simulink library "MixerLib"  (R2022b)
settings: Solver=VariableStepAuto  StartTime=0.0  StopTime=10.0  RelTol=1e-3
undefined symbols (not defined in the file or in its folder): maxGain
settings Model: Creator=ak1044356  LastModifiedBy=sa1045272
settings SolverCC: AlgebraicLoopSolver=TrustRegion
settings DebuggingCC: UnconnectedInputMsg=warning  UnconnectedOutputMsg=warning  UnconnectedLineMsg=warning  SFMachineParentedDataDiag=warning  ArithmeticOperatorsInVariantConditions=warning
settings ModelReferenceCC: EnableRefExpFcnMdlSchedulingChecks=on
settings SFSimCC: CustomCodeUndefinedFunction=UseInterfaceOnly

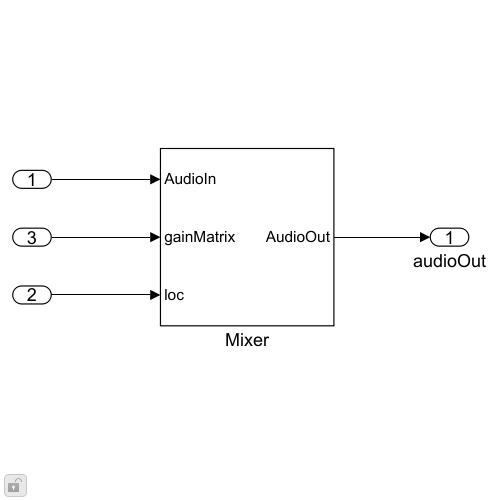
[thumbnail: Simulink's stored preview of the top-level diagram]
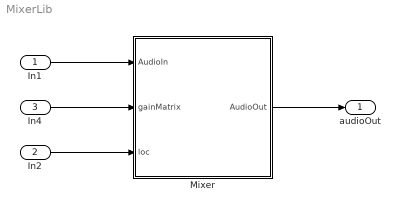
== system MixerLib ==
  In1 : Inport
  In2 : Inport  Port=2
  In4 : Inport  Port=3
  Mixer : Subsystem
  audioOut : Outport  VectorParamsAs1DForOutWhenUnconnected=off
  wires:
  Mixer/1(AudioOut) -> audioOut/1
  In1/1 -> Mixer/1(AudioIn)
  In2/1 -> Mixer/3(loc)
  In4/1 -> Mixer/2(gainMatrix)

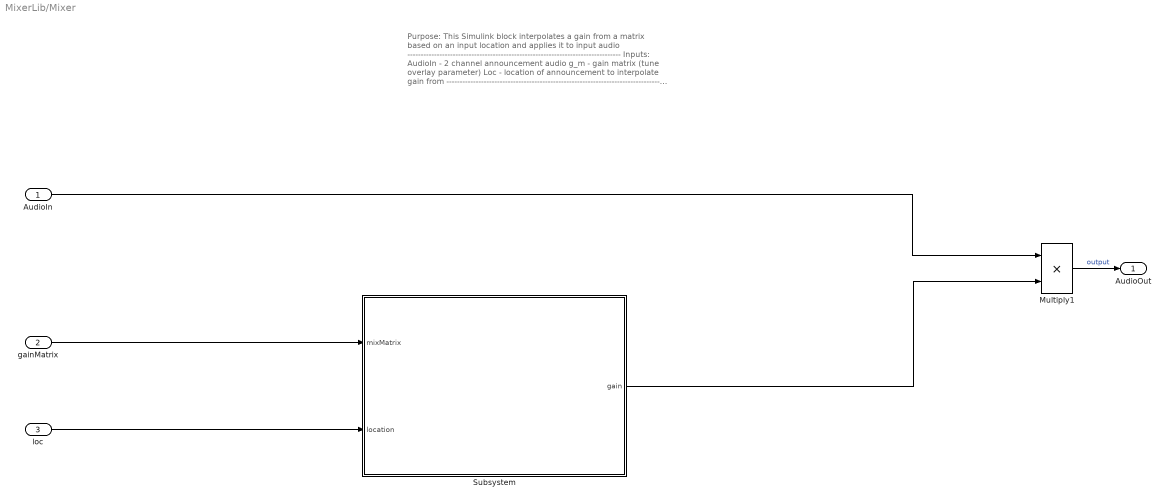
== system MixerLib/Mixer ==
  note: Purpose:
      | This Simulink block interpolates a gain from a matrix
      | based on an input location and applies it to input audio
      | --------------------------------------------------------------------------------
      | Inputs:
      | AudioIn - 2 channel announcement audio
      | g_m - gain matrix (tune overlay parameter)
      | Loc - location of announcement to interpolate gain from
      | --------------------------------------------------------------------------------
      | Outputs:
      | AudioOut - 2 channel announcement audio with applied gain
      | gain [temporary] - gain applied to audio, for debugging
  AudioIn : Inport  OutDataTypeStr=single
  gainMatrix : Inport  Port=2
  loc : Inport  Port=3
  Multiply1 : Product  OutDataTypeStr=single
  Subsystem : Subsystem
  AudioOut : Outport  VectorParamsAs1DForOutWhenUnconnected=off
  wires:
  AudioIn/1 -> Multiply1/1
  Multiply1/1 -> AudioOut/1  "output"
  gainMatrix/1 -> Subsystem/1(mixMatrix)
  Subsystem/1(gain) -> Multiply1/2
  loc/1 -> Subsystem/2(location)

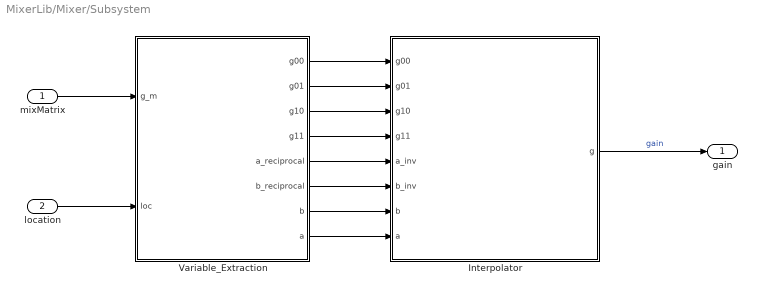
== system MixerLib/Mixer/Subsystem ==
  mixMatrix : Inport
  location : Inport  Port=2
  Interpolator : Subsystem
  Variable_Extraction : Subsystem
  gain : Outport  VectorParamsAs1DForOutWhenUnconnected=off
  wires:
  Interpolator/1(g) -> gain/1  "gain"
  mixMatrix/1 -> Variable_Extraction/1(g_m)
  Variable_Extraction/8(a) -> Interpolator/8(a)
  Variable_Extraction/4(g11) -> Interpolator/4(g11)
  Variable_Extraction/3(g10) -> Interpolator/3(g10)
  Variable_Extraction/2(g01) -> Interpolator/2(g01)
  location/1 -> Variable_Extraction/2(loc)
  Variable_Extraction/5(a_reciprocal) -> Interpolator/5(a_inv)
  Variable_Extraction/1(g00) -> Interpolator/1(g00)
  Variable_Extraction/6(b_reciprocal) -> Interpolator/6(b_inv)
  Variable_Extraction/7(b) -> Interpolator/7(b)

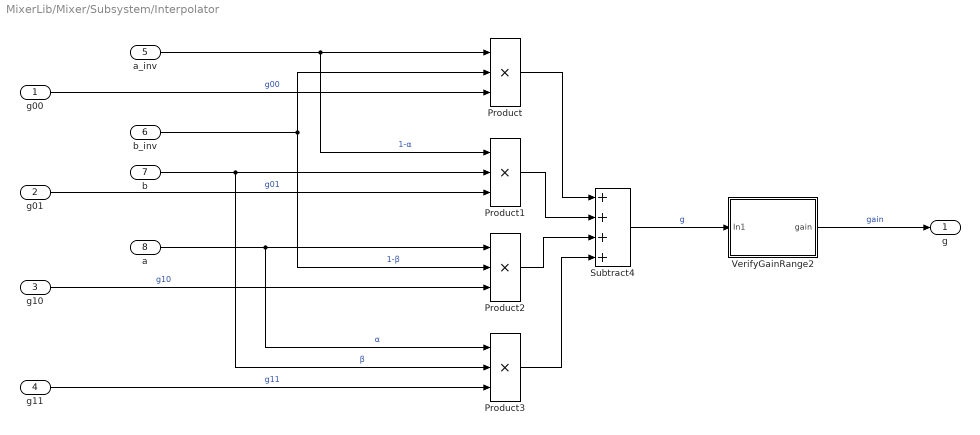
== system MixerLib/Mixer/Subsystem/Interpolator ==
  g00 : Inport
  g01 : Inport  Port=2
  g10 : Inport  Port=3
  g11 : Inport  Port=4
  a_inv : Inport  Port=5
  b_inv : Inport  Port=6
  b : Inport  Port=7
  a : Inport  Port=8
  Product{,1..3} (4 alike) : Product  Inputs=3  OutDataTypeStr=single
  Subtract4 : Sum  Inputs=++++  OutDataTypeStr=single
  VerifyGainRange2 : Subsystem
  g : Outport  VectorParamsAs1DForOutWhenUnconnected=off
  wires:
  g00/1 -> Product/3  "g00"
  Product1/1 -> Subtract4/2
  Product2/1 -> Subtract4/3
  Product3/1 -> Subtract4/4
  a/1 -> Product3/1, Product2/1  "α"
  a_inv/1 -> Product1/1, Product/1  "1-α"
  g10/1 -> Product2/3  "g10"
  b_inv/1 -> Product/2, Product2/2  "1-β"
  Subtract4/1 -> VerifyGainRange2/1(In1)  "g"
  b/1 -> Product1/2, Product3/2  "β"
  Product/1 -> Subtract4/1
  g11/1 -> Product3/3  "g11"
  g01/1 -> Product1/3  "g01"
  VerifyGainRange2/1(gain) -> g/1  "gain"

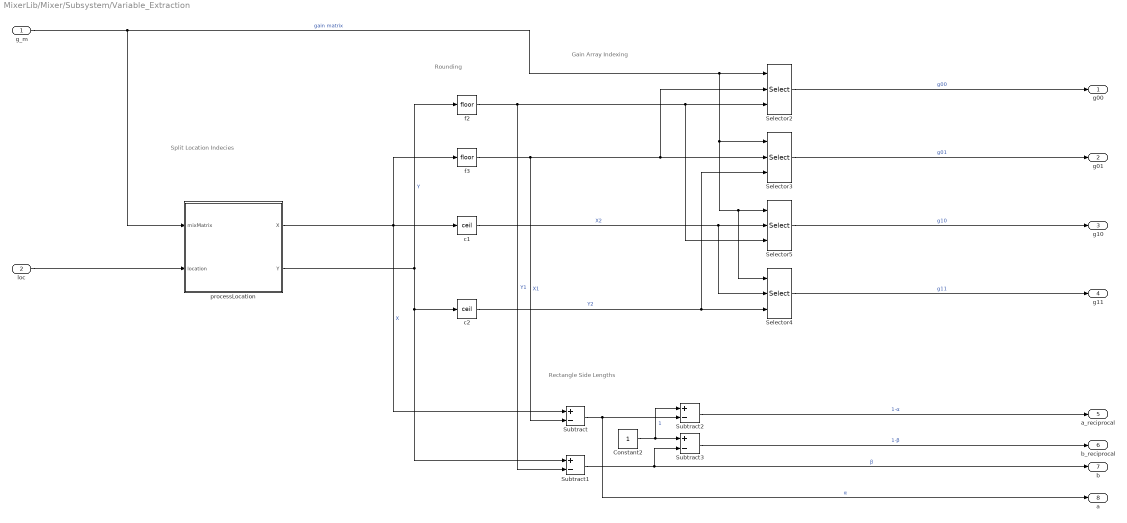
== system MixerLib/Mixer/Subsystem/Variable_Extraction ==
  note: Split Location Indecies
  note: Rectangle Side Lengths
  note: Rounding
  note: Gain Array Indexing
  g_m : Inport  OutDataTypeStr=single
  loc : Inport  Port=2
  Constant2 : Constant  OutDataTypeStr=single
  Selector{2..5} (4 alike) : Selector  NumberOfDimensions=2  InputPortWidth=2  IndexOptions=Index vector (port),Index vector (port)  Indices=[1 3],1  OutputSizes=1,1
  Subtract{,1..3} (4 alike) : Sum  Inputs=+-  OutDataTypeStr=single
  c1 : Rounding  Operator=ceil
  "c2 " : Rounding  Operator=ceil
  f2 : Rounding
  f3 : Rounding
  processLocation : Subsystem
  g00 : Outport  VectorParamsAs1DForOutWhenUnconnected=off
  g01 : Outport  Port=2  VectorParamsAs1DForOutWhenUnconnected=off
  g10 : Outport  Port=3  VectorParamsAs1DForOutWhenUnconnected=off
  g11 : Outport  Port=4  VectorParamsAs1DForOutWhenUnconnected=off
  a_reciprocal : Outport  Port=5  VectorParamsAs1DForOutWhenUnconnected=off
  b_reciprocal : Outport  Port=6  VectorParamsAs1DForOutWhenUnconnected=off
  b : Outport  Port=7  VectorParamsAs1DForOutWhenUnconnected=off
  a : Outport  Port=8  VectorParamsAs1DForOutWhenUnconnected=off
  wires:
  Subtract3/1 -> b_reciprocal/1  "1-β"
  Subtract2/1 -> a_reciprocal/1  "1-α"
  processLocation/2(Y) -> f2/1, Subtract1/1, "c2 "/1  "Y"
  Selector2/1 -> g00/1  "g00"
  Selector3/1 -> g01/1  "g01"
  Selector4/1 -> g11/1  "g11"
  Selector5/1 -> g10/1  "g10"
  Subtract/1 -> a/1, Subtract2/2  "α"
  g_m/1 -> processLocation/1(mixMatrix), Selector4/1, Selector5/1, Selector3/1, Selector2/1  "gain matrix"
  "c2 "/1 -> Selector3/3, Selector4/3  "Y2"
  f2/1 -> Subtract1/2, Selector5/3, Selector2/3  "Y1"
  Constant2/1 -> Subtract2/1, Subtract3/1  "1"
  f3/1 -> Selector3/2, Selector2/2, Subtract/2  "X1"
  c1/1 -> Selector4/2, Selector5/2  "X2"
  Subtract1/1 -> b/1, Subtract3/2  "β"
  processLocation/1(X) -> Subtract/1, f3/1, c1/1  "X"
  loc/1 -> processLocation/2(location)

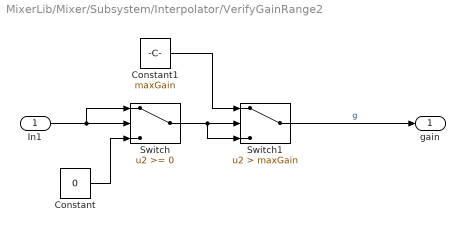
== system MixerLib/Mixer/Subsystem/Interpolator/VerifyGainRange2 ==
  In1 : Inport
  Constant : Constant  Value=0
  Constant1 : Constant  Value=maxGain
  Switch : Switch  SaturateOnIntegerOverflow=off  InputSameDT=off
  Switch1 : Switch  Criteria=u2 > Threshold  Threshold=maxGain  SaturateOnIntegerOverflow=off  InputSameDT=off
  gain : Outport  VectorParamsAs1DForOutWhenUnconnected=off
  wires:
  Switch/1 -> Switch1/3, Switch1/2
  Constant1/1 -> Switch1/1
  In1/1 -> Switch/1, Switch/2
  Switch1/1 -> gain/1  "g"
  Constant/1 -> Switch/3

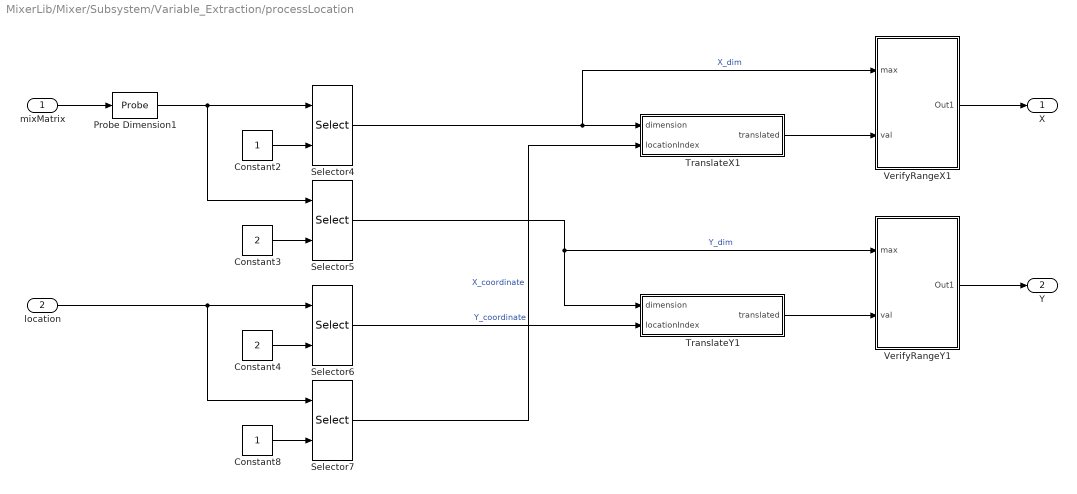
== system MixerLib/Mixer/Subsystem/Variable_Extraction/processLocation ==
  mixMatrix : Inport
  location : Inport  Port=2
  Constant2 : Constant  OutDataTypeStr=single
  Constant3 : Constant  Value=2  OutDataTypeStr=single
  Constant4 : Constant  Value=2  OutDataTypeStr=single
  Constant8 : Constant  OutDataTypeStr=single
  Probe Dimension1 : Probe  ProbeWidth=off  ProbeSampleTime=off  ProbeComplexSignal=off  ProbeSignalDimensions=on
  Selector{4..7} (4 alike) : Selector  InputPortWidth=2  IndexOptions=Index vector (port)  Indices=[1 3]  OutputSizes=1
  TranslateX1 : Subsystem
  TranslateY1 : Subsystem
  VerifyRangeX1 : Subsystem
  VerifyRangeY1 : Subsystem
  X : Outport  VectorParamsAs1DForOutWhenUnconnected=off
  Y : Outport  Port=2  VectorParamsAs1DForOutWhenUnconnected=off
  wires:
  Selector5/1 -> TranslateY1/1(dimension), VerifyRangeY1/1(max)  "Y_dim"
  Selector6/1 -> TranslateY1/2(locationIndex)  "Y_coordinate"
  Selector4/1 -> VerifyRangeX1/1(max), TranslateX1/1(dimension)  "X_dim"
  mixMatrix/1 -> Probe Dimension1/1
  Probe Dimension1/1 -> Selector5/1, Selector4/1
  Selector7/1 -> TranslateX1/2(locationIndex)  "X_coordinate"
  Constant3/1 -> Selector5/2
  location/1 -> Selector7/1, Selector6/1
  Constant4/1 -> Selector6/2
  Constant2/1 -> Selector4/2
  Constant8/1 -> Selector7/2
  TranslateY1/1(translated) -> VerifyRangeY1/2(val)
  TranslateX1/1(translated) -> VerifyRangeX1/2(val)
  VerifyRangeX1/1(Out1) -> X/1
  VerifyRangeY1/1(Out1) -> Y/1

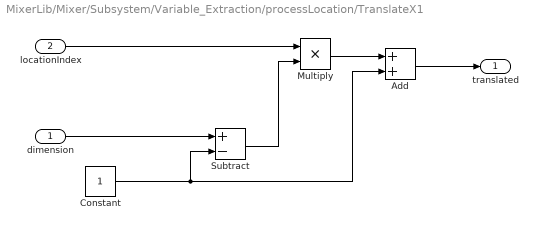
== system MixerLib/Mixer/Subsystem/Variable_Extraction/processLocation/TranslateX1 ==
  dimension : Inport
  locationIndex : Inport  Port=2
  Add : Sum
  Constant : Constant
  Multiply : Product
  Subtract : Sum  Inputs=+-
  translated : Outport  VectorParamsAs1DForOutWhenUnconnected=off
  wires:
  Constant/1 -> Add/2, Subtract/2
  dimension/1 -> Subtract/1
  Add/1 -> translated/1
  Multiply/1 -> Add/1
  Subtract/1 -> Multiply/2
  locationIndex/1 -> Multiply/1

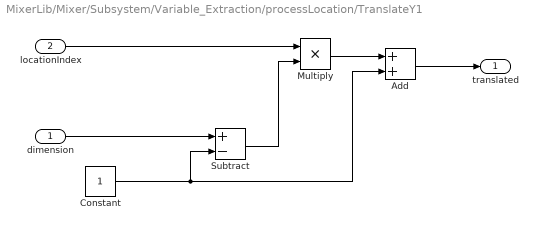
== system MixerLib/Mixer/Subsystem/Variable_Extraction/processLocation/TranslateY1 ==
  dimension : Inport
  locationIndex : Inport  Port=2
  Add : Sum
  Constant : Constant
  Multiply : Product
  Subtract : Sum  Inputs=+-
  translated : Outport  VectorParamsAs1DForOutWhenUnconnected=off
  wires:
  locationIndex/1 -> Multiply/1
  Subtract/1 -> Multiply/2
  Multiply/1 -> Add/1
  Add/1 -> translated/1
  dimension/1 -> Subtract/1
  Constant/1 -> Subtract/2, Add/2

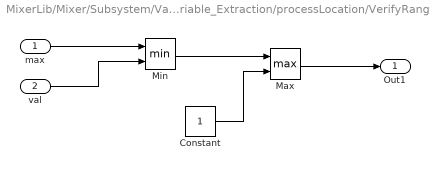
== system MixerLib/Mixer/Subsystem/Variable_Extraction/processLocation/VerifyRangeX1 ==
  max : Inport
  val : Inport  Port=2
  Constant : Constant
  Max : MinMax  Function=max  Inputs=2
  Min : MinMax  Inputs=2
  Out1 : Outport  VectorParamsAs1DForOutWhenUnconnected=off
  wires:
  Max/1 -> Out1/1
  Constant/1 -> Max/2
  Min/1 -> Max/1
  max/1 -> Min/1
  val/1 -> Min/2

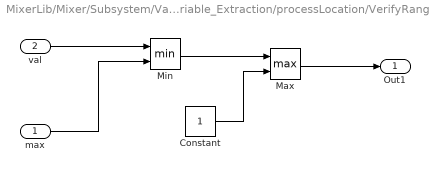
== system MixerLib/Mixer/Subsystem/Variable_Extraction/processLocation/VerifyRangeY1 ==
  max : Inport
  val : Inport  Port=2
  Constant : Constant
  Max : MinMax  Function=max  Inputs=2
  Min : MinMax  Inputs=2
  Out1 : Outport  VectorParamsAs1DForOutWhenUnconnected=off
  wires:
  Max/1 -> Out1/1
  Constant/1 -> Max/2
  Min/1 -> Max/1
  max/1 -> Min/2
  val/1 -> Min/1
